simulink model "exp1"  (R2022a)
settings: Solver=ode45  StartTime=0.0  StopTime=20.0  RelTol=1e-3
settings Model: Creator=Guilherme  LastModifiedBy=Guilherme

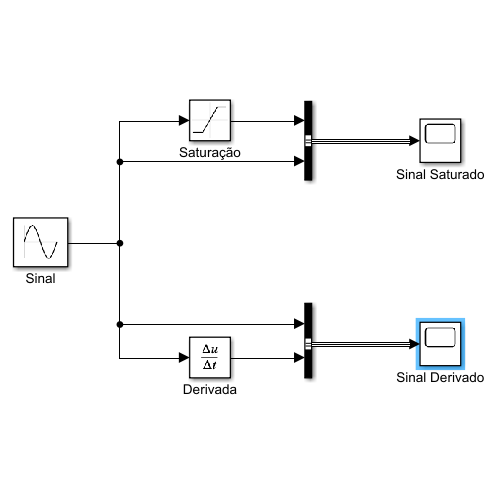
[thumbnail: Simulink's stored preview of the top-level diagram]
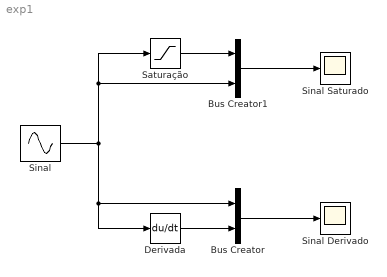
== system exp1 ==
  Bus Creator : BusCreator  Inputs=2
  Bus Creator1 : BusCreator  Inputs=2
  Derivada : Derivative
  Saturação : Saturate  UpperLimit=1  LowerLimit=-1
  Sinal : Sin  Amplitude=2  SampleTime=0
  Sinal Derivado : Scope
  Sinal Saturado : Scope
  wires:
  Sinal/1 -> Bus Creator/1, Derivada/1, Bus Creator1/2, Saturação/1
  Saturação/1 -> Bus Creator1/1
  Derivada/1 -> Bus Creator/2
  Bus Creator/1 -> Sinal Derivado/1
  Bus Creator1/1 -> Sinal Saturado/1
